simulink model "CDPR_simulation"  (R2021b)
settings: Solver=VariableStepAuto  StartTime=0.0  StopTime=40.0  RelTol=1e-3
values from neighbouring files (symbols this model uses):
  a = [-2.0 2.0 ... (first row only)    [init.m]
  A_p = [0  1   0  0   0  0 ... (first row only)    [init.m]
  b = [-0.05  0.05 ... (first row only)    [init.m]
  B_p = [0     0     0 ... (first row only)    [init.m]
  Clarke = 2/3*[1 -1/2       -1/2 ... (first row only)    [motor_init.m]
  epsilon_1 = 1e-17    [init.m]
  epsilon_2 = 1e-17    [init.m]
  f_max = 60*ones(m,1)    [init.m]
  f_min = 2*ones(m,1)    [init.m]
  f_ref = 0.5*(f_min+f_max)    [init.m]
  fourier_coeff_a = [ 0.08333    0.00000     0.00000 ... (first row only)    [motor_init.m]
  fourier_coeff_b = [-1.23020    0.60792     0.60792 ... (first row only)    [motor_init.m]
  J_m_inv = 1000*1/J_m    (= 41564.487302)    [motor_init.m]
  K_e = 0.052    [motor_init.m]
  k_spring = diag(200*ones(m,1))    [init.m]
  k_spring_inv = inv(k_spring)    [init.m]
  l_0 = inverseKinematics(a, b, x, m)    [init.m]
  L_m = 8.97e-6    (= 8.97e-06)    [motor_init.m]
  m = 4    [init.m]
  n_pole_pairs = n_poles/2    (= 7)    [motor_init.m]
  R_m = 19.00e-3    (= 0.019)    [motor_init.m]
  r_winch = 60.0e-3    (= 0.06)    [init.m]
  tau = 1e-6    (= 1e-06)    [init.m]
  theta_r_0 = (l_0-k_spring_inv*f_ref)/r_winch    [init.m]
  x_0 = [x(1); 0; x(2); 0; x(3);0]    [init.m]
  xi = 2    [init.m]
(part 1 of 2)
settings Model: Creator=Sølve  LastModifiedBy=Sølve

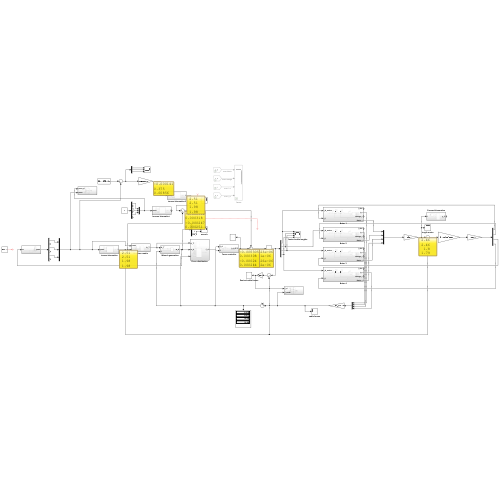
[thumbnail: Simulink's stored preview of the top-level diagram]
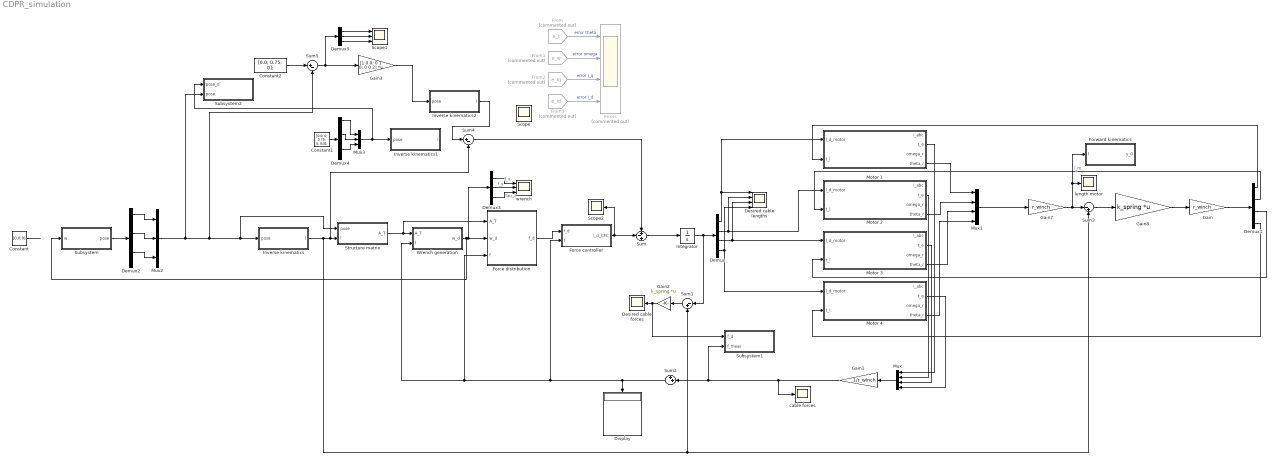
== system CDPR_simulation ==
  Constant : Constant  Value=[0;0;0]
  Constant1 : Constant  Value=[0.0; 0; 0.75; 0; 0;0];
  Constant2 : Constant  Value=[0.0; 0.75; 0];
  Demux : Demux
  Demux1 : Demux
  Demux2 : Demux  Outputs=6
  Demux3 : Demux  Outputs=3
  Demux4 : Demux  Outputs=6
  Demux5 : Demux  Outputs=3
  Desired cable forces : Scope
  Desired cable lengths : Scope  NumInputPorts=4
  Display : Display
      settings: Decimation=3
  Errors : Scope  Commented=on  NumInputPorts=4
  Force controller : Subsystem
  Force distribution : Subsystem
  Forward kinematics : Subsystem
  From : From  Commented=on  GotoTag=e_t  TagVisibility=global
  From1 : From  Commented=on  GotoTag=e_w  TagVisibility=global
  From2 : From  Commented=on  GotoTag=e_iq  TagVisibility=global
  From3 : From  Commented=on  GotoTag=e_id  TagVisibility=global
  Gain : Gain  Gain=r_winch
  Gain1 : Gain  Gain=1/r_winch
  Gain2 : Gain  Gain=k_spring  Multiplication=Matrix(K*u) (u vector)
  Gain3 : Gain  Gain=[1 0 0; 0 1 0; 0 0 2]  Multiplication=Matrix(K*u) (u vector)
  Gain7 : Gain  Gain=r_winch
  Gain8 : Gain  Gain=k_spring  Multiplication=Matrix(K*u) (u vector)
  Integrator : Integrator  InitialCondition=l_0-k_spring_inv*f_ref
  Inverse kinematics : Subsystem
  Inverse kinematics1 : Subsystem
  Inverse kinematics2 : Subsystem
  Motor 1 : Subsystem
  Motor 2 : Subsystem
  Motor 3 : Subsystem
  Motor 4 : Subsystem
  Mux : Mux
  Mux1 : Mux
  Mux2 : Mux  Inputs=3
  Mux3 : Mux  Inputs=3
  Scope : Scope
  Scope1 : Scope  NumInputPorts=3
  Scope2 : Scope
  Structure matrix : Subsystem
  Subsystem : Subsystem
  Subsystem1 : Subsystem
  Subsystem2 : Subsystem
  Sum : Sum  Inputs=+-+
  Sum1 : Sum  Inputs=|-+
  Sum2 : Sum  Inputs=++|
  Sum3 : Sum  Inputs=|-+
  Sum4 : Sum  Inputs=|+-
  Sum5 : Sum  Inputs=|+-
  Wrench generation : Subsystem
  cable forces : Scope
  length motor : Scope
  wrench : Scope  NumInputPorts=3
  wires:
  Mux2/1 -> Subsystem2/2(pose), Sum5/2, Structure matrix/1(pose), Inverse kinematics/1(pose)
  Constant/1 -> ?
  Structure matrix/1(A_T) -> Force distribution/1(A_T), Wrench generation/1(A_T)
  Wrench generation/1(w_d) -> Subsystem/1(w), Force distribution/2(w_d), Demux3/1
  Force controller/1(l_d_CFC) -> Sum/2, Scope2/1
  From3/1 -> Errors/4  "error i_d"
  From2/1 -> Errors/3  "error i_q"
  From/1 -> Errors/1  "error theta"
  From1/1 -> Errors/2  "error omega"
  Sum/1 -> Integrator/1
  Demux/1 -> Desired cable lengths/1, Motor 1/1(l_d_motor)
  Motor 1/4(theta_r) -> Mux1/1
  Sum2/1 -> Force controller/2(f), Force distribution/3(f), Wrench generation/2(f), Display/1
  Demux3/1 -> wrench/1  "f_x"
  Demux3/2 -> wrench/2  "f_y"
  Demux3/3 -> wrench/3  "tau_z"
  Demux/2 -> Motor 2/1(l_d_motor), Desired cable lengths/2
  Mux1/1 -> Gain7/1
  Motor 2/4(theta_r) -> Mux1/2
  Gain7/1 -> length motor/1, Forward kinematics/1(l), Sum3/1  "l_m"
  Motor 3/4(theta_r) -> Mux1/3
  Demux/3 -> Motor 3/1(l_d_motor), Desired cable lengths/3
  Demux/4 -> Motor 4/1(l_d_motor), Desired cable lengths/4
  Motor 4/4(theta_r) -> Mux1/4
  Sum3/1 -> Gain8/1
  Inverse kinematics/1(l) -> Sum1/2, Sum3/2, Sum4/2, Structure matrix/2(l)
  Gain8/1 -> Gain/1
  Gain/1 -> Demux1/1
  Demux1/1 -> Motor 1/2(t_l)
  Demux1/2 -> Motor 2/2(t_l)
  Demux1/3 -> Motor 3/2(t_l)
  Demux1/4 -> Motor 4/2(t_l)
  Motor 1/2(t_e) -> Mux/1
  Motor 2/2(t_e) -> Mux/2
  Motor 3/2(t_e) -> Mux/3
  Motor 4/2(t_e) -> Mux/4
  Mux/1 -> Gain1/1
  Force distribution/1(f_d) -> Force controller/1(f_d)
  Gain1/1 -> cable forces/1, Subsystem1/2(f_meas), Sum2/2
  Integrator/1 -> Sum1/1, Demux/1
  Subsystem/1(pose) -> Demux2/1
  Demux2/1 -> Mux2/1
  Demux2/3 -> Mux2/2
  Demux2/5 -> Mux2/3
  Gain2/1 -> Subsystem1/1(f_d), Desired cable forces/1
  Sum1/1 -> Gain2/1
  Constant1/1 -> Demux4/1
  Inverse kinematics2/1(l) -> Sum4/1
  Sum4/1 -> Sum/1
  Demux4/1 -> Mux3/1
  Demux4/3 -> Mux3/2
  Demux4/5 -> Mux3/3
  Mux3/1 -> Subsystem2/1(pose_d), Inverse kinematics1/1(pose)
  Constant2/1 -> Sum5/1
  Sum5/1 -> Gain3/1, Demux5/1
  Demux5/1 -> Scope1/1
  Demux5/2 -> Scope1/2
  Demux5/3 -> Scope1/3
  Gain3/1 -> Inverse kinematics2/1(pose)
  ? -> ?

== system CDPR_simulation/Force controller ==
  f_d : Inport
  f : Inport  Port=2
  Gain : Gain  Gain=5
  Gain1 : Gain  Gain=k_spring_inv  Multiplication=Matrix(K*u) (u vector)
  Gain2 : Gain  Gain=2
  Integrator : Integrator
  Sum : Sum  Inputs=|+-
  Sum1 : Sum  Inputs=++|
  l_d_CFC : Outport
  wires:
  f_d/1 -> Sum/1
  f/1 -> Sum/2
  Sum/1 -> Integrator/1, Gain/1
  Gain/1 -> Sum1/2
  Gain1/1 -> l_d_CFC/1
  Integrator/1 -> Gain2/1
  Gain2/1 -> ?
  Sum1/1 -> Gain1/1

== system CDPR_simulation/Force distribution ==
  A_T : Inport
  w_d : Inport  Port=2
  f : Inport  Port=3
  Constant : Constant  Commented=on  Value=f_min
  Constant1 : Constant  Commented=on  Value=f_max
  Constant2 : Constant  Value=f_min
  Constant3 : Constant  Value=f_max
  Constant4 : Constant  Value=f_ref
  Constant5 : Constant  Value=m
  Force distribution calculation : MATLAB Function  TreatAsAtomicUnit=on
  MATLAB Function : MATLAB Function  Commented=on  TreatAsAtomicUnit=on
  f_d : Outport
  wires:
  A_T/1 -> Force distribution calculation/1(A_T)
  Force distribution calculation/1(f_d) -> f_d/1
  Constant1/1 -> MATLAB Function/4(f_max)
  Constant/1 -> MATLAB Function/3(f_min)
  w_d/1 -> Force distribution calculation/6(w)
  Constant2/1 -> Force distribution calculation/3(f_min)
  Constant3/1 -> Force distribution calculation/4(f_max)
  Constant4/1 -> Force distribution calculation/5(f_ref)
  Constant5/1 -> Force distribution calculation/7(m)
  f/1 -> Force distribution calculation/2(f)

== system CDPR_simulation/Forward kinematics ==
  l : Inport
  Constant : Constant  Value=b
  Constant1 : Constant  Value=a
  Constant2 : Constant  Value=m
  Constant3 : Constant  Value=tau
  Constant4 : Constant  Value=epsilon_1
  Constant5 : Constant  Value=epsilon_2
  Constant6 : Constant  Value=xi
  MATLAB Function : MATLAB Function  TreatAsAtomicUnit=on
  MATLAB Function1 : MATLAB Function  TreatAsAtomicUnit=on
  y_0 : Outport
  wires:
  l/1 -> MATLAB Function1/3(l), MATLAB Function/4(l)
  Constant/1 -> MATLAB Function1/2(b), MATLAB Function/2(b)
  Constant1/1 -> MATLAB Function1/1(a), MATLAB Function/1(a)
  MATLAB Function1/1(y_0) -> MATLAB Function/3(y_0)
  Constant2/1 -> MATLAB Function/9(m)
  MATLAB Function/1(y_i) -> y_0/1
  Constant3/1 -> MATLAB Function/5(tau)
  Constant5/1 -> MATLAB Function/7(epsilon_2)
  Constant4/1 -> MATLAB Function/6(epsilon_1)
  Constant6/1 -> MATLAB Function/8(xi)

== system CDPR_simulation/Inverse kinematics ==
  pose : Inport
  Constant2 : Constant  Value=m
  Distal anchor points : Constant  Value=b
  Inverse kinematics : MATLAB Function  TreatAsAtomicUnit=on
  Proximal anchor points : Constant  Value=a
  l : Outport
  wires:
  Constant2/1 -> Inverse kinematics/4(m)
  Proximal anchor points/1 -> Inverse kinematics/1(a)
  Inverse kinematics/1(l) -> l/1
  Distal anchor points/1 -> Inverse kinematics/2(b)
  pose/1 -> Inverse kinematics/3(pose)

== system CDPR_simulation/Inverse kinematics1 ==
  pose : Inport
  Constant2 : Constant  Value=m
  Distal anchor points : Constant  Value=b
  Inverse kinematics : MATLAB Function  TreatAsAtomicUnit=on
  Proximal anchor points : Constant  Value=a
  l : Outport
  wires:
  pose/1 -> Inverse kinematics/3(pose)
  Distal anchor points/1 -> Inverse kinematics/2(b)
  Inverse kinematics/1(l) -> l/1
  Proximal anchor points/1 -> Inverse kinematics/1(a)
  Constant2/1 -> Inverse kinematics/4(m)

== system CDPR_simulation/Inverse kinematics2 ==
  pose : Inport
  Constant2 : Constant  Value=m
  Distal anchor points : Constant  Value=b
  Inverse kinematics : MATLAB Function  TreatAsAtomicUnit=on
  Proximal anchor points : Constant  Value=a
  l : Outport
  wires:
  Constant2/1 -> Inverse kinematics/4(m)
  Proximal anchor points/1 -> Inverse kinematics/1(a)
  Inverse kinematics/1(l) -> l/1
  Distal anchor points/1 -> Inverse kinematics/2(b)
  pose/1 -> Inverse kinematics/3(pose)

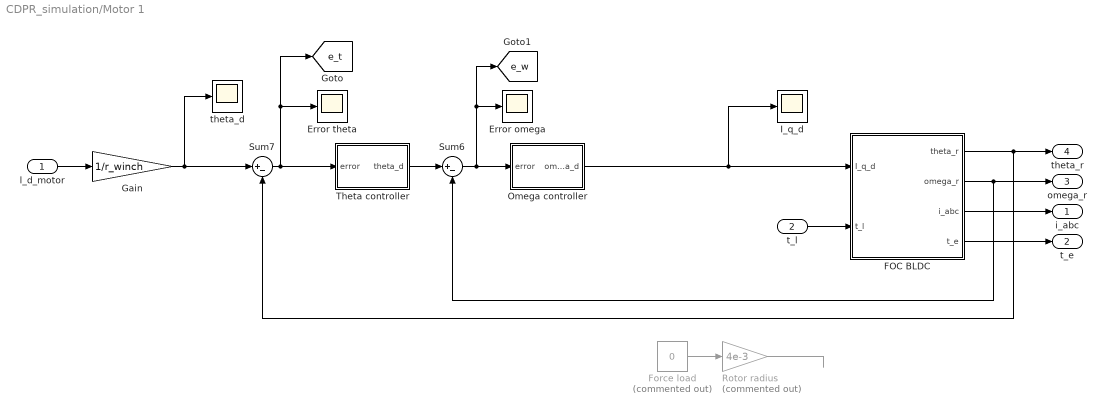
== system CDPR_simulation/Motor 1 ==
  l_d_motor : Inport
  t_l : Inport  Port=2
  Error omega : Scope
  Error theta : Scope
  FOC BLDC : Subsystem
  Force load : Constant  Commented=on  Value=0
  Gain : Gain  Gain=1/r_winch
  I_q_d : Scope
  Omega controller : Subsystem
  Rotor radius : Gain  Commented=on  Gain=4e-3
  Sum6 : Sum  Inputs=|+-
  Sum7 : Sum  Inputs=|+-
  Theta controller : Subsystem
  theta_d : Scope
  i_abc : Outport
  t_e : Outport  Port=2
  omega_r : Outport  Port=3
  theta_r : Outport  Port=4
  tag scope: e_t=global, e_w=global
  wires:
  FOC BLDC/2(omega_r) -> omega_r/1, Sum6/2
  FOC BLDC/3(i_abc) -> i_abc/1
  Sum7/1 -> Theta controller/1(error), [e_t], Error theta/1
  Sum6/1 -> Omega controller/1(error), Error omega/1, [e_w]
  Force load/1 -> Rotor radius/1
  FOC BLDC/1(theta_r) -> theta_r/1, Sum7/2
  Rotor radius/1 -> ?
  Theta controller/1(theta_d) -> Sum6/1
  FOC BLDC/4(t_e) -> t_e/1
  Omega controller/1(omega_d) -> I_q_d/1, FOC BLDC/1(I_q_d)
  l_d_motor/1 -> Gain/1
  t_l/1 -> FOC BLDC/2(t_l)
  Gain/1 -> theta_d/1, Sum7/1

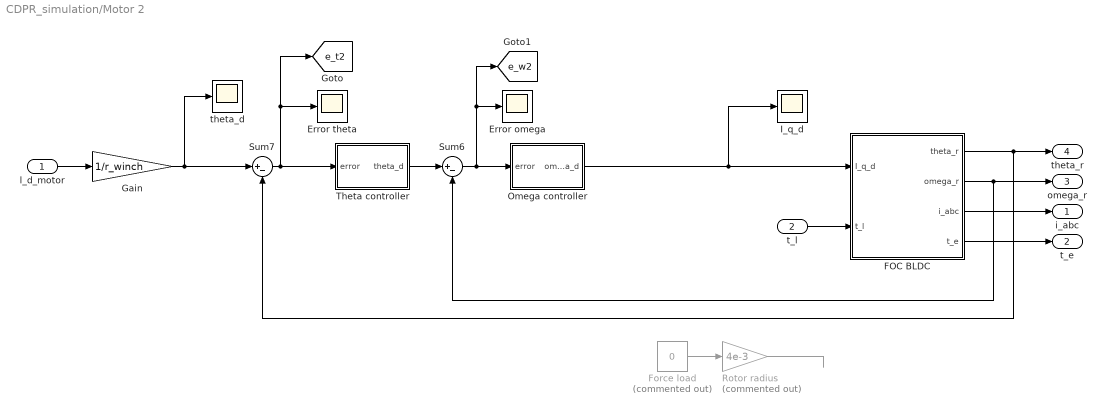
== system CDPR_simulation/Motor 2 ==
  l_d_motor : Inport
  t_l : Inport  Port=2
  Error omega : Scope
  Error theta : Scope
  FOC BLDC : Subsystem
  Force load : Constant  Commented=on  Value=0
  Gain : Gain  Gain=1/r_winch
  I_q_d : Scope
  Omega controller : Subsystem
  Rotor radius : Gain  Commented=on  Gain=4e-3
  Sum6 : Sum  Inputs=|+-
  Sum7 : Sum  Inputs=|+-
  Theta controller : Subsystem
  theta_d : Scope
  i_abc : Outport
  t_e : Outport  Port=2
  omega_r : Outport  Port=3
  theta_r : Outport  Port=4
  tag scope: e_t2=global, e_w2=global
  wires:
  Gain/1 -> Sum7/1, theta_d/1
  t_l/1 -> FOC BLDC/2(t_l)
  l_d_motor/1 -> Gain/1
  Omega controller/1(omega_d) -> FOC BLDC/1(I_q_d), I_q_d/1
  FOC BLDC/4(t_e) -> t_e/1
  Theta controller/1(theta_d) -> Sum6/1
  Rotor radius/1 -> ?
  FOC BLDC/1(theta_r) -> Sum7/2, theta_r/1
  Force load/1 -> Rotor radius/1
  Sum6/1 -> [e_w2], Error omega/1, Omega controller/1(error)
  Sum7/1 -> Error theta/1, [e_t2], Theta controller/1(error)
  FOC BLDC/3(i_abc) -> i_abc/1
  FOC BLDC/2(omega_r) -> Sum6/2, omega_r/1

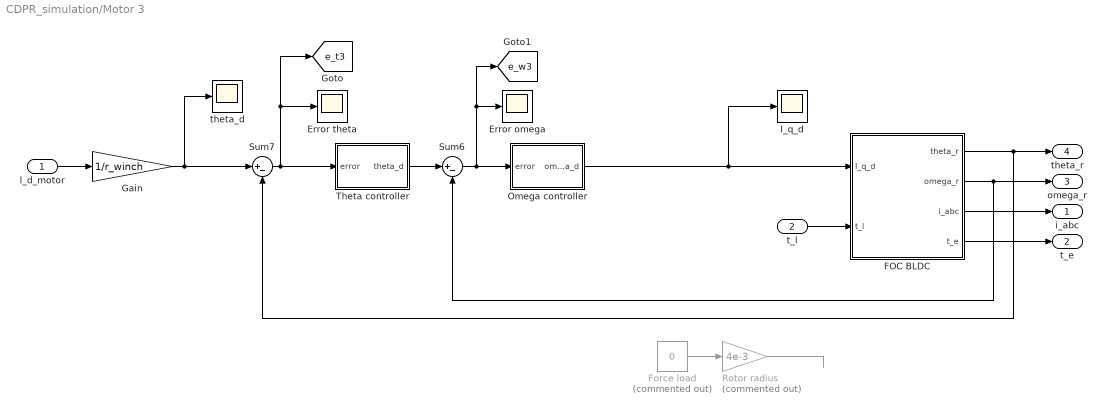
== system CDPR_simulation/Motor 3 ==
  l_d_motor : Inport
  t_l : Inport  Port=2
  Error omega : Scope
  Error theta : Scope
  FOC BLDC : Subsystem
  Force load : Constant  Commented=on  Value=0
  Gain : Gain  Gain=1/r_winch
  I_q_d : Scope
  Omega controller : Subsystem
  Rotor radius : Gain  Commented=on  Gain=4e-3
  Sum6 : Sum  Inputs=|+-
  Sum7 : Sum  Inputs=|+-
  Theta controller : Subsystem
  theta_d : Scope
  i_abc : Outport
  t_e : Outport  Port=2
  omega_r : Outport  Port=3
  theta_r : Outport  Port=4
  tag scope: e_t3=global, e_w3=global
  wires:
  FOC BLDC/2(omega_r) -> omega_r/1, Sum6/2
  FOC BLDC/3(i_abc) -> i_abc/1
  Sum7/1 -> Theta controller/1(error), [e_t3], Error theta/1
  Sum6/1 -> Omega controller/1(error), Error omega/1, [e_w3]
  Force load/1 -> Rotor radius/1
  FOC BLDC/1(theta_r) -> theta_r/1, Sum7/2
  Rotor radius/1 -> ?
  Theta controller/1(theta_d) -> Sum6/1
  FOC BLDC/4(t_e) -> t_e/1
  Omega controller/1(omega_d) -> I_q_d/1, FOC BLDC/1(I_q_d)
  l_d_motor/1 -> Gain/1
  t_l/1 -> FOC BLDC/2(t_l)
  Gain/1 -> theta_d/1, Sum7/1

== system CDPR_simulation/Motor 4 ==
  l_d_motor : Inport
  t_l : Inport  Port=2
  Error omega : Scope
  Error theta : Scope
  FOC BLDC : Subsystem
  Force load : Constant  Commented=on  Value=0
  Gain : Gain  Gain=1/r_winch
  I_q_d : Scope
  Omega controller : Subsystem
  Rotor radius : Gain  Commented=on  Gain=4e-3
  Sum6 : Sum  Inputs=|+-
  Sum7 : Sum  Inputs=|+-
  Theta controller : Subsystem
  theta_d : Scope
  i_abc : Outport
  t_e : Outport  Port=2
  omega_r : Outport  Port=3
  theta_r : Outport  Port=4
  tag scope: e_t4=global, e_w4=global
  wires:
  Gain/1 -> Sum7/1, theta_d/1
  t_l/1 -> FOC BLDC/2(t_l)
  l_d_motor/1 -> Gain/1
  Omega controller/1(omega_d) -> FOC BLDC/1(I_q_d), I_q_d/1
  FOC BLDC/4(t_e) -> t_e/1
  Theta controller/1(theta_d) -> Sum6/1
  Rotor radius/1 -> ?
  FOC BLDC/1(theta_r) -> Sum7/2, theta_r/1
  Force load/1 -> Rotor radius/1
  Sum6/1 -> [e_w4], Error omega/1, Omega controller/1(error)
  Sum7/1 -> Error theta/1, [e_t4], Theta controller/1(error)
  FOC BLDC/3(i_abc) -> i_abc/1
  FOC BLDC/2(omega_r) -> Sum6/2, omega_r/1

== system CDPR_simulation/Structure matrix ==
  pose : Inport
  l : Inport  Port=2
  Constant : Constant  Value=a
  Constant1 : Constant  Value=b
  Constant2 : Constant  Value=m
  MATLAB Function : MATLAB Function  TreatAsAtomicUnit=on
  Structure matrix calculation : MATLAB Function  TreatAsAtomicUnit=on
  A_T : Outport
  wires:
  pose/1 -> Structure matrix calculation/2(pose), MATLAB Function/3(pose)
  Constant1/1 -> Structure matrix calculation/3(b), MATLAB Function/2(b)
  Constant/1 -> MATLAB Function/1(a)
  MATLAB Function/1(u) -> Structure matrix calculation/1(u)
  Structure matrix calculation/1(A_T) -> A_T/1
  l/1 -> MATLAB Function/4(l_ik)
  Constant2/1 -> Structure matrix calculation/4(m), MATLAB Function/5(m)

== system CDPR_simulation/Subsystem ==
  w : Inport
  Demux : Demux  Outputs=6
  Gain : Gain  Gain=B_p  Multiplication=Matrix(K*u) (u vector)
  Gain1 : Gain  Gain=A_p  Multiplication=Matrix(K*u) (u vector)
  Integrator : Integrator  InitialCondition=x_0
  Mux : Mux  Inputs=6
  Scope : Scope  NumInputPorts=3
  Sum : Sum  Inputs=|++
  XY Graph : Record  FileSettingsInternal="{\"entries\":[{\"content\":{\"excelSettings\":{\"content\":{},\"type\":\"Streamout.ExcelSettings\"}},\"type\":\"Streamout.FileSettingStorage\",\"uuid\":\"53abfe96-87d4-4a9b-ba96-94057390cc17\"}],\"packageUris\":[\"http://schema.mathworks.com/mf0/streamout_blocks/R2020a\"],\"version\":\"1.0\"}"  Layout=[1 1]  SignalsInternal="{\"entries\":[{\"content\":{\"signals\":[{\"content\":{\"blockPath\":[\"CDPR_simulation/Subsystem/XY Graph\"],\"channel\":[],\"dimensions\":[1],\"domain\":\"CDPR_simulation/Subsystem/XY Graph\",\"lineColor\":\"#a2142f\",\"plots\":[1],\"port\":1,\"sid\":[\"\"],\"signalID\":17344,\"signalName\":\"Demux:1\"},\"type\":\"RecordBlkView.Signal\",\"uuid\":\"32875e08-411f-4073-9301-21440afacdc0\"},{\"content\":{\"blockPath\":[\"CDPR_simulation/Subsystem/XY Graph\"],\"channel\":[],\"dimensions\":[1],\"domain\":\"CDPR_simulation/Subsystem/XY Graph\",\"lineColor\":\"#139fff\",\"plots\":[1],\"port\":2,\"sid\":[\"\"],\"signalID\":17348,\"signalName\":\"Demux:3\"},\"type\":\"RecordBlkView.Signal\",\"uuid\":\"bdc768ac-4432-491c-a3b0-f805c164fc47\"}]},\"type\":\"RecordBlkView.InputSignals\",\"uuid\":\"dc717eb6-7a39-403c-b8e2-f99afc544a76\"}],\"packageUris\":[\"http://schema.mathworks.com/mf0/streamout_blocks/R2020a\"],\"version\":\"1.0\"}"  VisualizationBindings="{\"xyplotplugin\":{\"info\":[{\"series\":[{\"bindingParametersList\":[{\"parameter\":\"X-Axis\",\"signalID\":17344,\"signalName\":\"Demux:1\"},{\"parameter\":\"Y-Axis\",\"signalID\":17348,\"signalName\":\"Demux:3\"}],\"seriesID\":4472}],\"subplotID\":1}]}}"  CompatibilityTag=XY
  pose : Outport
  wires:
  w/1 -> Gain/1
  Gain/1 -> Sum/1
  Sum/1 -> Integrator/1
  Gain1/1 -> Sum/2
  Integrator/1 -> Demux/1, Gain1/1
  Demux/1 -> XY Graph/1, Scope/1, Mux/1
  Demux/3 -> Scope/2, XY Graph/2, Mux/3
  Demux/5 -> Scope/3, Mux/5
  Mux/1 -> pose/1
  Demux/2 -> Mux/2
  Demux/4 -> Mux/4
  Demux/6 -> Mux/6

== system CDPR_simulation/Subsystem1 ==
  f_d : Inport
  f_meas : Inport  Port=2
  Demux : Demux
  Demux1 : Demux
  Desired v. measured cable forces : Scope  NumInputPorts=4
  Mux{,1..3} (4 alike) : Mux  Inputs=2
  wires:
  f_d/1 -> Demux/1
  f_meas/1 -> Demux1/1
  Demux/1 -> Mux/1  "Desired force cable 1"
  Demux1/1 -> Mux/2  "Measured force cable 1"
  Demux/2 -> Mux1/1  "Desired force cable 2"
  Demux1/2 -> Mux1/2  "Measured force cable 2"
  Demux/3 -> Mux2/1  "Desired force cable 3"
  Demux1/3 -> Mux2/2  "Measured force cable 3"
  Demux/4 -> Mux3/1  "Desired force cable 4"
  Demux1/4 -> Mux3/2  "Measured force cable 4"
  Mux/1 -> Desired v. measured cable forces/1
  Mux1/1 -> Desired v. measured cable forces/2
  Mux2/1 -> Desired v. measured cable forces/3
  Mux3/1 -> Desired v. measured cable forces/4

== system CDPR_simulation/Subsystem2 ==
  pose_d : Inport
  pose : Inport  Port=2
  Demux : Demux  Outputs=3
  Demux1 : Demux  Outputs=3
  Desired v. actual pose : Scope  NumInputPorts=3
  Mux : Mux  Inputs=2
  Mux1 : Mux  Inputs=2
  Mux2 : Mux  Inputs=2
  wires:
  pose_d/1 -> Demux/1
  pose/1 -> Demux1/1
  Demux/1 -> Mux/1  "Desired x-coord"
  Demux1/1 -> Mux/2  "Actual x-coord"
  Demux/2 -> Mux1/1  "Desired y-coord"
  Demux1/2 -> Mux1/2  "Actual y-coord"
  Demux1/3 -> Mux2/2  "Actual angle"
  Demux/3 -> Mux2/1  "Desired angle"
  Mux/1 -> Desired v. actual pose/1
  Mux1/1 -> Desired v. actual pose/2
  Mux2/1 -> Desired v. actual pose/3

== system CDPR_simulation/Wrench generation ==
  A_T : Inport
  f : Inport  Port=2
  Gain : Gain
  Matrix Multiply : Product  Multiplication=Matrix(*)
  w_d : Outport
  wires:
  A_T/1 -> Gain/1
  f/1 -> Matrix Multiply/2
  Gain/1 -> Matrix Multiply/1
  Matrix Multiply/1 -> w_d/1

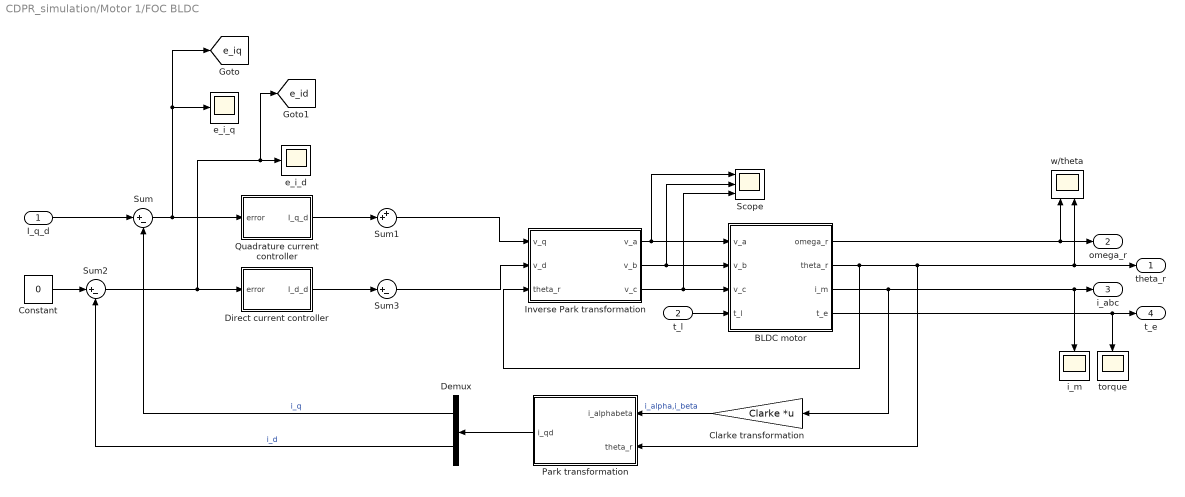
== system CDPR_simulation/Motor 1/FOC BLDC ==
  I_q_d : Inport
  t_l : Inport  Port=2
  BLDC motor : Subsystem
  Clarke transformation : Gain  Gain=Clarke  Multiplication=Matrix(K*u) (u vector)
  Constant : Constant  Value=0
  Demux : Demux  Outputs=2
  Direct current controller : Subsystem
  Inverse Park transformation : MATLAB Function  TreatAsAtomicUnit=on
  Park transformation : MATLAB Function  TreatAsAtomicUnit=on
  Quadrature current controller : Subsystem
  Scope : Scope  NumInputPorts=3
  Sum : Sum  Inputs=|+-
  Sum1 : Sum  Inputs=++|
  Sum2 : Sum  Inputs=|+-
  Sum3 : Sum  Inputs=|+-
  e_i_d : Scope
  e_i_q : Scope
  i_m : Scope
  torque : Scope
  w/theta : Scope  NumInputPorts=2
  theta_r : Outport
  omega_r : Outport  Port=2
  i_abc : Outport  Port=3
  t_e : Outport  Port=4
  tag scope: e_id=global, e_iq=global
  wires:
  Sum/1 -> Quadrature current controller/1(error), [e_iq], e_i_q/1
  Quadrature current controller/1(I_q_d) -> Sum1/2
  Constant/1 -> Sum2/1
  Sum2/1 -> Direct current controller/1(error), [e_id], e_i_d/1
  Direct current controller/1(I_d_d) -> Sum3/1
  Sum1/1 -> Inverse Park transformation/1(v_q)
  Sum3/1 -> Inverse Park transformation/2(v_d)
  Inverse Park transformation/1(v_a) -> Scope/1, BLDC motor/1(v_a)
  Inverse Park transformation/2(v_b) -> Scope/2, BLDC motor/2(v_b)
  Inverse Park transformation/3(v_c) -> Scope/3, BLDC motor/3(v_c)
  t_l/1 -> BLDC motor/4(t_l)
  BLDC motor/1(omega_r) -> omega_r/1, w/theta/1
  Clarke transformation/1 -> Park transformation/1(i_alphabeta)  "i_alpha,i_beta"
  BLDC motor/2(theta_r) -> Park transformation/2(theta_r), theta_r/1, w/theta/2, Inverse Park transformation/3(theta_r)
  Park transformation/1(i_qd) -> Demux/1
  Demux/1 -> Sum/2  "i_q"
  Demux/2 -> Sum2/2  "i_d"
  BLDC motor/3(i_m) -> i_m/1, i_abc/1, Clarke transformation/1
  BLDC motor/4(t_e) -> torque/1, t_e/1
  I_q_d/1 -> Sum/1

== system CDPR_simulation/Motor 1/Omega controller ==
  error : Inport
  Gain : Gain  Gain=30
  Gain1 : Gain  Gain=120
  Gain2 : Gain  Gain=30
  Gain3 : Gain  Gain=70
  Integrator : Integrator
  Sum : Sum  Inputs=++|
  omega_d : Outport
  wires:
  Sum/1 -> omega_d/1
  Gain/1 -> Sum/1
  Gain1/1 -> Sum/2
  Integrator/1 -> Gain1/1
  error/1 -> Integrator/1, Gain/1

== system CDPR_simulation/Motor 1/Theta controller ==
  error : Inport
  Gain : Gain  Gain=10
  Gain1 : Gain  Gain=30
  Gain2 : Gain  Gain=0.2
  Gain3 : Gain  Gain=15
  Integrator : Integrator
  Sum : Sum  Inputs=++|
  theta_d : Outport
  wires:
  error/1 -> Gain/1, Integrator/1
  Integrator/1 -> Gain1/1
  Gain1/1 -> Sum/2
  Gain/1 -> Sum/1
  Sum/1 -> theta_d/1

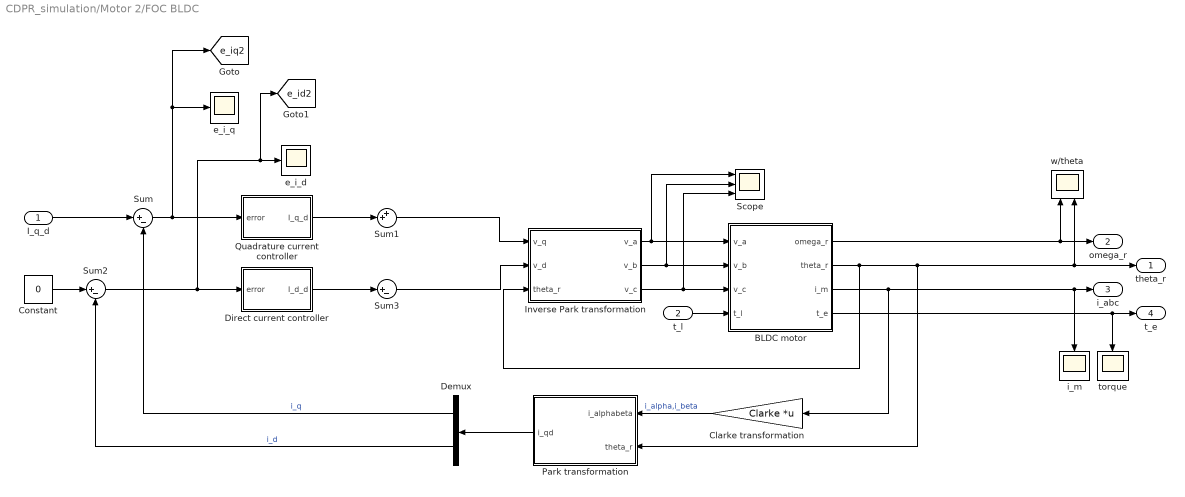
== system CDPR_simulation/Motor 2/FOC BLDC ==
  I_q_d : Inport
  t_l : Inport  Port=2
  BLDC motor : Subsystem
  Clarke transformation : Gain  Gain=Clarke  Multiplication=Matrix(K*u) (u vector)
  Constant : Constant  Value=0
  Demux : Demux  Outputs=2
  Direct current controller : Subsystem
  Inverse Park transformation : MATLAB Function  TreatAsAtomicUnit=on
  Park transformation : MATLAB Function  TreatAsAtomicUnit=on
  Quadrature current controller : Subsystem
  Scope : Scope  NumInputPorts=3
  Sum : Sum  Inputs=|+-
  Sum1 : Sum  Inputs=++|
  Sum2 : Sum  Inputs=|+-
  Sum3 : Sum  Inputs=|+-
  e_i_d : Scope
  e_i_q : Scope
  i_m : Scope
  torque : Scope
  w/theta : Scope  NumInputPorts=2
  theta_r : Outport
  omega_r : Outport  Port=2
  i_abc : Outport  Port=3
  t_e : Outport  Port=4
  tag scope: e_id2=global, e_iq2=global
  wires:
  I_q_d/1 -> Sum/1
  BLDC motor/4(t_e) -> t_e/1, torque/1
  BLDC motor/3(i_m) -> Clarke transformation/1, i_abc/1, i_m/1
  Demux/2 -> Sum2/2  "i_d"
  Demux/1 -> Sum/2  "i_q"
  Park transformation/1(i_qd) -> Demux/1
  BLDC motor/2(theta_r) -> Inverse Park transformation/3(theta_r), w/theta/2, theta_r/1, Park transformation/2(theta_r)
  Clarke transformation/1 -> Park transformation/1(i_alphabeta)  "i_alpha,i_beta"
  BLDC motor/1(omega_r) -> w/theta/1, omega_r/1
  t_l/1 -> BLDC motor/4(t_l)
  Inverse Park transformation/3(v_c) -> BLDC motor/3(v_c), Scope/3
  Inverse Park transformation/2(v_b) -> BLDC motor/2(v_b), Scope/2
  Inverse Park transformation/1(v_a) -> BLDC motor/1(v_a), Scope/1
  Sum3/1 -> Inverse Park transformation/2(v_d)
  Sum1/1 -> Inverse Park transformation/1(v_q)
  Direct current controller/1(I_d_d) -> Sum3/1
  Sum2/1 -> e_i_d/1, [e_id2], Direct current controller/1(error)
  Constant/1 -> Sum2/1
  Quadrature current controller/1(I_q_d) -> Sum1/2
  Sum/1 -> e_i_q/1, [e_iq2], Quadrature current controller/1(error)

== system CDPR_simulation/Motor 2/Omega controller ==
  error : Inport
  Gain : Gain  Gain=30
  Gain1 : Gain  Gain=120
  Gain2 : Gain  Gain=30
  Gain3 : Gain  Gain=70
  Integrator : Integrator
  Sum : Sum  Inputs=++|
  omega_d : Outport
  wires:
  error/1 -> Gain/1, Integrator/1
  Integrator/1 -> Gain1/1
  Gain1/1 -> Sum/2
  Gain/1 -> Sum/1
  Sum/1 -> omega_d/1

== system CDPR_simulation/Motor 2/Theta controller ==
  error : Inport
  Gain : Gain  Gain=10
  Gain1 : Gain  Gain=30
  Gain2 : Gain  Gain=0.2
  Gain3 : Gain  Gain=15
  Integrator : Integrator
  Sum : Sum  Inputs=++|
  theta_d : Outport
  wires:
  Sum/1 -> theta_d/1
  Gain/1 -> Sum/1
  Gain1/1 -> Sum/2
  Integrator/1 -> Gain1/1
  error/1 -> Integrator/1, Gain/1

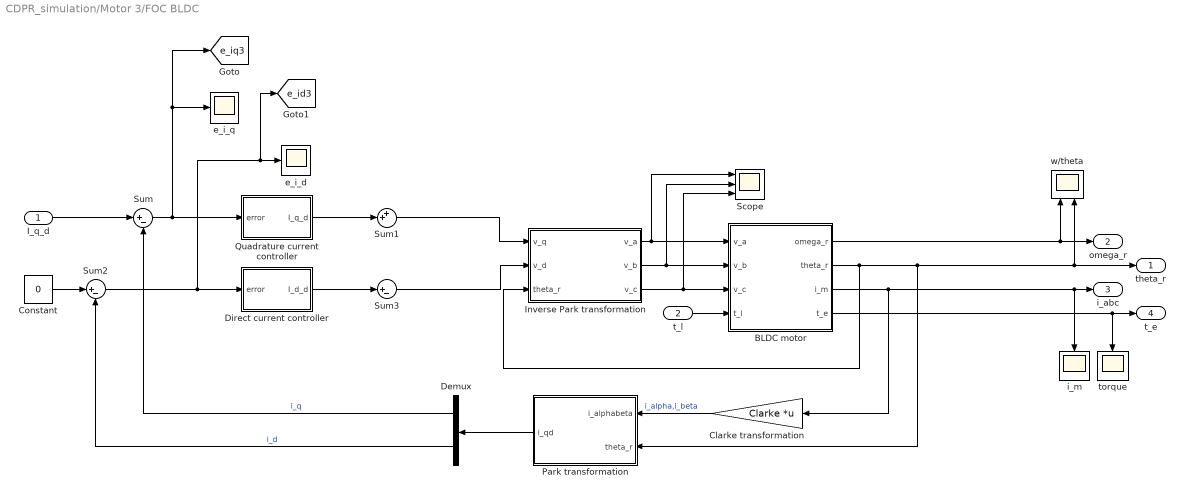
== system CDPR_simulation/Motor 3/FOC BLDC ==
  I_q_d : Inport
  t_l : Inport  Port=2
  BLDC motor : Subsystem
  Clarke transformation : Gain  Gain=Clarke  Multiplication=Matrix(K*u) (u vector)
  Constant : Constant  Value=0
  Demux : Demux  Outputs=2
  Direct current controller : Subsystem
  Inverse Park transformation : MATLAB Function  TreatAsAtomicUnit=on
  Park transformation : MATLAB Function  TreatAsAtomicUnit=on
  Quadrature current controller : Subsystem
  Scope : Scope  NumInputPorts=3
  Sum : Sum  Inputs=|+-
  Sum1 : Sum  Inputs=++|
  Sum2 : Sum  Inputs=|+-
  Sum3 : Sum  Inputs=|+-
  e_i_d : Scope
  e_i_q : Scope
  i_m : Scope
  torque : Scope
  w/theta : Scope  NumInputPorts=2
  theta_r : Outport
  omega_r : Outport  Port=2
  i_abc : Outport  Port=3
  t_e : Outport  Port=4
  tag scope: e_id3=global, e_iq3=global
  wires:
  Sum/1 -> Quadrature current controller/1(error), [e_iq3], e_i_q/1
  Quadrature current controller/1(I_q_d) -> Sum1/2
  Constant/1 -> Sum2/1
  Sum2/1 -> Direct current controller/1(error), [e_id3], e_i_d/1
  Direct current controller/1(I_d_d) -> Sum3/1
  Sum1/1 -> Inverse Park transformation/1(v_q)
  Sum3/1 -> Inverse Park transformation/2(v_d)
  Inverse Park transformation/1(v_a) -> Scope/1, BLDC motor/1(v_a)
  Inverse Park transformation/2(v_b) -> Scope/2, BLDC motor/2(v_b)
  Inverse Park transformation/3(v_c) -> Scope/3, BLDC motor/3(v_c)
  t_l/1 -> BLDC motor/4(t_l)
  BLDC motor/1(omega_r) -> omega_r/1, w/theta/1
  Clarke transformation/1 -> Park transformation/1(i_alphabeta)  "i_alpha,i_beta"
  BLDC motor/2(theta_r) -> Park transformation/2(theta_r), theta_r/1, w/theta/2, Inverse Park transformation/3(theta_r)
  Park transformation/1(i_qd) -> Demux/1
  Demux/1 -> Sum/2  "i_q"
  Demux/2 -> Sum2/2  "i_d"
  BLDC motor/3(i_m) -> i_m/1, i_abc/1, Clarke transformation/1
  BLDC motor/4(t_e) -> torque/1, t_e/1
  I_q_d/1 -> Sum/1

== system CDPR_simulation/Motor 3/Omega controller ==
  error : Inport
  Gain : Gain  Gain=30
  Gain1 : Gain  Gain=120
  Gain2 : Gain  Gain=30
  Gain3 : Gain  Gain=70
  Integrator : Integrator
  Sum : Sum  Inputs=++|
  omega_d : Outport
  wires:
  Sum/1 -> omega_d/1
  Gain/1 -> Sum/1
  Gain1/1 -> Sum/2
  Integrator/1 -> Gain1/1
  error/1 -> Integrator/1, Gain/1

== system CDPR_simulation/Motor 3/Theta controller ==
  error : Inport
  Gain : Gain  Gain=10
  Gain1 : Gain  Gain=30
  Gain2 : Gain  Gain=0.2
  Gain3 : Gain  Gain=15
  Integrator : Integrator
  Sum : Sum  Inputs=++|
  theta_d : Outport
  wires:
  error/1 -> Gain/1, Integrator/1
  Integrator/1 -> Gain1/1
  Gain1/1 -> Sum/2
  Gain/1 -> Sum/1
  Sum/1 -> theta_d/1

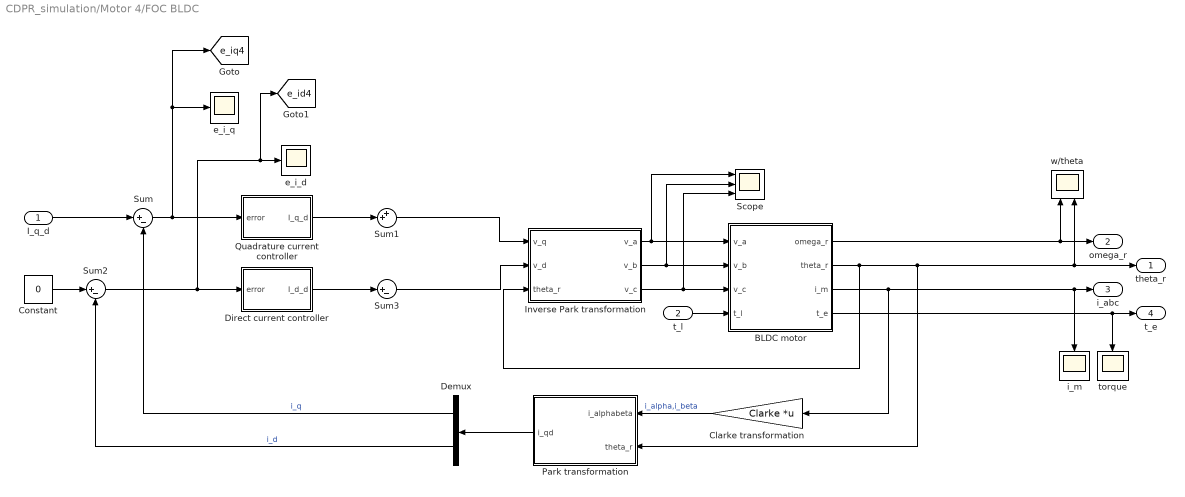
== system CDPR_simulation/Motor 4/FOC BLDC ==
  I_q_d : Inport
  t_l : Inport  Port=2
  BLDC motor : Subsystem
  Clarke transformation : Gain  Gain=Clarke  Multiplication=Matrix(K*u) (u vector)
  Constant : Constant  Value=0
  Demux : Demux  Outputs=2
  Direct current controller : Subsystem
  Inverse Park transformation : MATLAB Function  TreatAsAtomicUnit=on
  Park transformation : MATLAB Function  TreatAsAtomicUnit=on
  Quadrature current controller : Subsystem
  Scope : Scope  NumInputPorts=3
  Sum : Sum  Inputs=|+-
  Sum1 : Sum  Inputs=++|
  Sum2 : Sum  Inputs=|+-
  Sum3 : Sum  Inputs=|+-
  e_i_d : Scope
  e_i_q : Scope
  i_m : Scope
  torque : Scope
  w/theta : Scope  NumInputPorts=2
  theta_r : Outport
  omega_r : Outport  Port=2
  i_abc : Outport  Port=3
  t_e : Outport  Port=4
  tag scope: e_id4=global, e_iq4=global
  wires:
  I_q_d/1 -> Sum/1
  BLDC motor/4(t_e) -> t_e/1, torque/1
  BLDC motor/3(i_m) -> Clarke transformation/1, i_abc/1, i_m/1
  Demux/2 -> Sum2/2  "i_d"
  Demux/1 -> Sum/2  "i_q"
  Park transformation/1(i_qd) -> Demux/1
  BLDC motor/2(theta_r) -> Inverse Park transformation/3(theta_r), w/theta/2, theta_r/1, Park transformation/2(theta_r)
  Clarke transformation/1 -> Park transformation/1(i_alphabeta)  "i_alpha,i_beta"
  BLDC motor/1(omega_r) -> w/theta/1, omega_r/1
  t_l/1 -> BLDC motor/4(t_l)
  Inverse Park transformation/3(v_c) -> BLDC motor/3(v_c), Scope/3
  Inverse Park transformation/2(v_b) -> BLDC motor/2(v_b), Scope/2
  Inverse Park transformation/1(v_a) -> BLDC motor/1(v_a), Scope/1
  Sum3/1 -> Inverse Park transformation/2(v_d)
  Sum1/1 -> Inverse Park transformation/1(v_q)
  Direct current controller/1(I_d_d) -> Sum3/1
  Sum2/1 -> e_i_d/1, [e_id4], Direct current controller/1(error)
  Constant/1 -> Sum2/1
  Quadrature current controller/1(I_q_d) -> Sum1/2
  Sum/1 -> e_i_q/1, [e_iq4], Quadrature current controller/1(error)

== system CDPR_simulation/Motor 4/Omega controller ==
  error : Inport
  Gain : Gain  Gain=30
  Gain1 : Gain  Gain=120
  Gain2 : Gain  Gain=30
  Gain3 : Gain  Gain=70
  Integrator : Integrator
  Sum : Sum  Inputs=++|
  omega_d : Outport
  wires:
  error/1 -> Gain/1, Integrator/1
  Integrator/1 -> Gain1/1
  Gain1/1 -> Sum/2
  Gain/1 -> Sum/1
  Sum/1 -> omega_d/1

== system CDPR_simulation/Motor 4/Theta controller ==
  error : Inport
  Gain : Gain  Gain=10
  Gain1 : Gain  Gain=30
  Gain2 : Gain  Gain=0.2
  Gain3 : Gain  Gain=15
  Integrator : Integrator
  Sum : Sum  Inputs=++|
  theta_d : Outport
  wires:
  Sum/1 -> theta_d/1
  Gain/1 -> Sum/1
  Gain1/1 -> Sum/2
  Integrator/1 -> Gain1/1
  error/1 -> Integrator/1, Gain/1

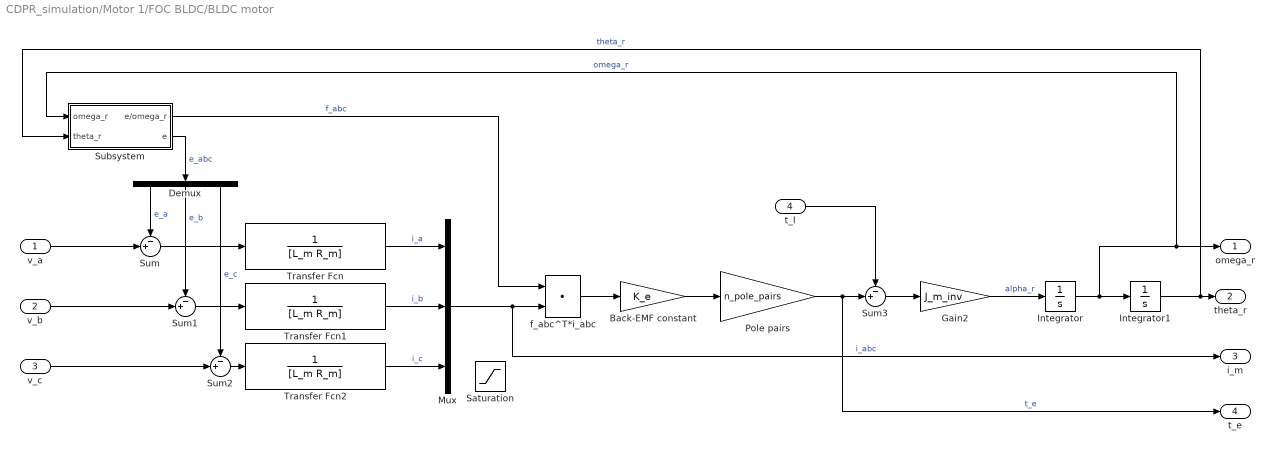
== system CDPR_simulation/Motor 1/FOC BLDC/BLDC motor ==
  v_a : Inport
  v_b : Inport  Port=2
  v_c : Inport  Port=3
  t_l : Inport  Port=4
  Back-EMF constant : Gain  Gain=K_e
  Demux : Demux  Outputs=3
  Gain2 : Gain  Gain=J_m_inv
  Integrator : Integrator  InitialCondition=0.001
  Integrator1 : Integrator  InitialCondition=theta_r_0(1)
  Mux : Mux  Inputs=3
  Pole pairs : Gain  Gain=n_pole_pairs
  Saturation : Saturate  UpperLimit=20  LowerLimit=20
  Subsystem : Subsystem
  Sum{,1..3} (4 alike) : Sum  Inputs=-+|
  Transfer Fcn : TransferFcn  Denominator=[L_m R_m]
  Transfer Fcn1 : TransferFcn  Denominator=[L_m R_m]
  Transfer Fcn2 : TransferFcn  Denominator=[L_m R_m]
  f_abc^T*i_abc : DotProduct  InputSameDT=on  OutDataTypeStr=Inherit: Inherit via internal rule
  omega_r : Outport
  theta_r : Outport  Port=2
  i_m : Outport  Port=3
  t_e : Outport  Port=4
  wires:
  v_a/1 -> Sum/2
  v_b/1 -> Sum1/2
  v_c/1 -> Sum2/2
  Demux/1 -> Sum/1  "e_a"
  Demux/2 -> Sum1/1  "e_b"
  Demux/3 -> Sum2/1  "e_c"
  Subsystem/2(e) -> Demux/1  "e_abc"
  Sum/1 -> Transfer Fcn/1
  Sum1/1 -> Transfer Fcn1/1
  Sum2/1 -> Transfer Fcn2/1
  Transfer Fcn2/1 -> Mux/3  "i_c"
  Transfer Fcn1/1 -> Mux/2  "i_b"
  Transfer Fcn/1 -> Mux/1  "i_a"
  Subsystem/1(e/omega_r) -> f_abc^T*i_abc/1  "f_abc"
  Sum3/1 -> Gain2/1
  f_abc^T*i_abc/1 -> Back-EMF constant/1
  Back-EMF constant/1 -> Pole pairs/1
  t_l/1 -> Sum3/1
  Gain2/1 -> Integrator/1  "alpha_r"
  Integrator/1 -> Subsystem/1(omega_r), omega_r/1, Integrator1/1  "omega_r"
  Integrator1/1 -> Subsystem/2(theta_r), theta_r/1  "theta_r"
  Pole pairs/1 -> t_e/1, Sum3/2  "t_e"
  Mux/1 -> f_abc^T*i_abc/2, i_m/1  "i_abc"

== system CDPR_simulation/Motor 1/FOC BLDC/Direct current controller ==
  error : Inport
  Gain : Gain  Gain=100
  Gain1 : Gain  Gain=70
  Integrator : Integrator
  Sum : Sum  Inputs=++|
  I_d_d : Outport
  wires:
  error/1 -> Gain/1, Integrator/1
  Integrator/1 -> Gain1/1
  Gain1/1 -> Sum/2
  Gain/1 -> Sum/1
  Sum/1 -> I_d_d/1

== system CDPR_simulation/Motor 1/FOC BLDC/Quadrature current controller ==
  error : Inport
  Gain : Gain  Gain=35
  Gain1 : Gain  Gain=50
  Integrator : Integrator
  Sum : Sum  Inputs=++|
  I_q_d : Outport
  wires:
  Sum/1 -> I_q_d/1
  Gain/1 -> Sum/1
  Gain1/1 -> Sum/2
  Integrator/1 -> Gain1/1
  error/1 -> Integrator/1, Gain/1

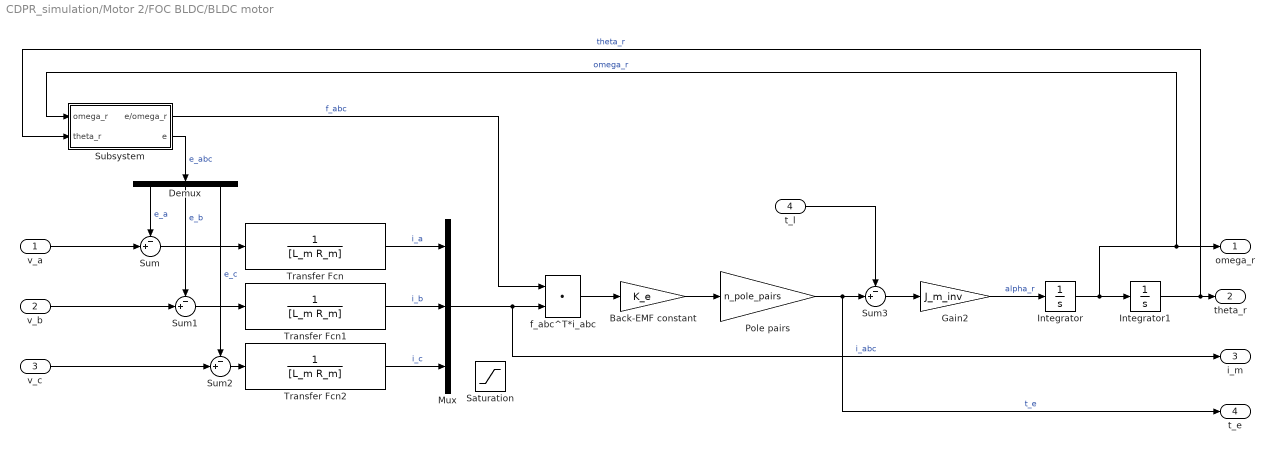
== system CDPR_simulation/Motor 2/FOC BLDC/BLDC motor ==
  v_a : Inport
  v_b : Inport  Port=2
  v_c : Inport  Port=3
  t_l : Inport  Port=4
  Back-EMF constant : Gain  Gain=K_e
  Demux : Demux  Outputs=3
  Gain2 : Gain  Gain=J_m_inv
  Integrator : Integrator  InitialCondition=0.001
  Integrator1 : Integrator  InitialCondition=theta_r_0(2)
  Mux : Mux  Inputs=3
  Pole pairs : Gain  Gain=n_pole_pairs
  Saturation : Saturate  UpperLimit=20  LowerLimit=20
  Subsystem : Subsystem
  Sum{,1..3} (4 alike) : Sum  Inputs=-+|
  Transfer Fcn : TransferFcn  Denominator=[L_m R_m]
  Transfer Fcn1 : TransferFcn  Denominator=[L_m R_m]
  Transfer Fcn2 : TransferFcn  Denominator=[L_m R_m]
  f_abc^T*i_abc : DotProduct  InputSameDT=on  OutDataTypeStr=Inherit: Inherit via internal rule
  omega_r : Outport
  theta_r : Outport  Port=2
  i_m : Outport  Port=3
  t_e : Outport  Port=4
  wires:
  Mux/1 -> i_m/1, f_abc^T*i_abc/2  "i_abc"
  Pole pairs/1 -> Sum3/2, t_e/1  "t_e"
  Integrator1/1 -> theta_r/1, Subsystem/2(theta_r)  "theta_r"
  Integrator/1 -> Integrator1/1, omega_r/1, Subsystem/1(omega_r)  "omega_r"
  Gain2/1 -> Integrator/1  "alpha_r"
  t_l/1 -> Sum3/1
  Back-EMF constant/1 -> Pole pairs/1
  f_abc^T*i_abc/1 -> Back-EMF constant/1
  Sum3/1 -> Gain2/1
  Subsystem/1(e/omega_r) -> f_abc^T*i_abc/1  "f_abc"
  Transfer Fcn/1 -> Mux/1  "i_a"
  Transfer Fcn1/1 -> Mux/2  "i_b"
  Transfer Fcn2/1 -> Mux/3  "i_c"
  Sum2/1 -> Transfer Fcn2/1
  Sum1/1 -> Transfer Fcn1/1
  Sum/1 -> Transfer Fcn/1
  Subsystem/2(e) -> Demux/1  "e_abc"
  Demux/3 -> Sum2/1  "e_c"
  Demux/2 -> Sum1/1  "e_b"
  Demux/1 -> Sum/1  "e_a"
  v_c/1 -> Sum2/2
  v_b/1 -> Sum1/2
  v_a/1 -> Sum/2

== system CDPR_simulation/Motor 2/FOC BLDC/Direct current controller ==
  error : Inport
  Gain : Gain  Gain=100
  Gain1 : Gain  Gain=70
  Integrator : Integrator
  Sum : Sum  Inputs=++|
  I_d_d : Outport
  wires:
  Sum/1 -> I_d_d/1
  Gain/1 -> Sum/1
  Gain1/1 -> Sum/2
  Integrator/1 -> Gain1/1
  error/1 -> Integrator/1, Gain/1

== system CDPR_simulation/Motor 2/FOC BLDC/Quadrature current controller ==
  error : Inport
  Gain : Gain  Gain=35
  Gain1 : Gain  Gain=50
  Integrator : Integrator
  Sum : Sum  Inputs=++|
  I_q_d : Outport
  wires:
  error/1 -> Gain/1, Integrator/1
  Integrator/1 -> Gain1/1
  Gain1/1 -> Sum/2
  Gain/1 -> Sum/1
  Sum/1 -> I_q_d/1

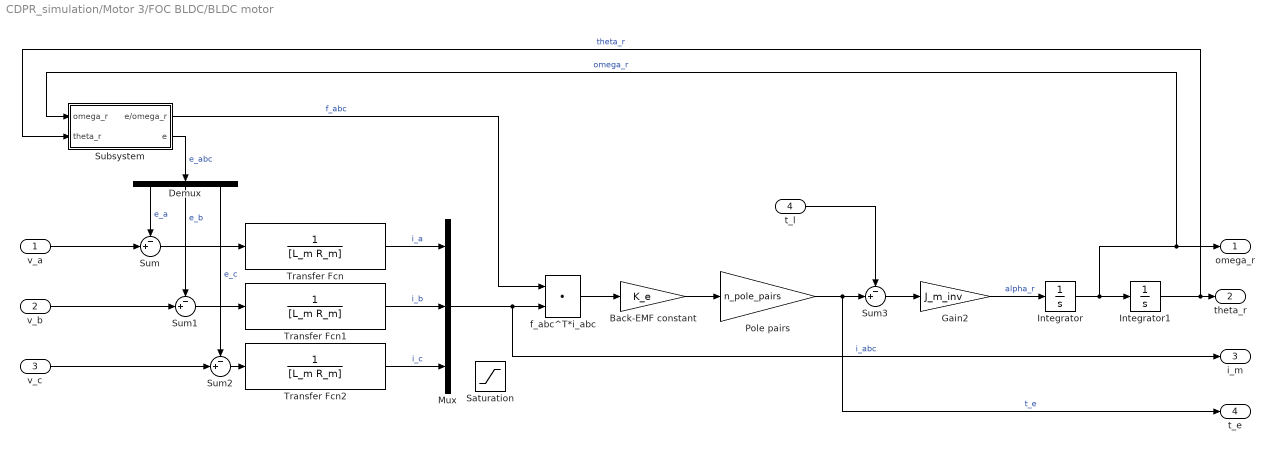
== system CDPR_simulation/Motor 3/FOC BLDC/BLDC motor ==
  v_a : Inport
  v_b : Inport  Port=2
  v_c : Inport  Port=3
  t_l : Inport  Port=4
  Back-EMF constant : Gain  Gain=K_e
  Demux : Demux  Outputs=3
  Gain2 : Gain  Gain=J_m_inv
  Integrator : Integrator  InitialCondition=0.001
  Integrator1 : Integrator  InitialCondition=theta_r_0(3)
  Mux : Mux  Inputs=3
  Pole pairs : Gain  Gain=n_pole_pairs
  Saturation : Saturate  UpperLimit=20  LowerLimit=20
  Subsystem : Subsystem
  Sum{,1..3} (4 alike) : Sum  Inputs=-+|
  Transfer Fcn : TransferFcn  Denominator=[L_m R_m]
  Transfer Fcn1 : TransferFcn  Denominator=[L_m R_m]
  Transfer Fcn2 : TransferFcn  Denominator=[L_m R_m]
  f_abc^T*i_abc : DotProduct  InputSameDT=on  OutDataTypeStr=Inherit: Inherit via internal rule
  omega_r : Outport
  theta_r : Outport  Port=2
  i_m : Outport  Port=3
  t_e : Outport  Port=4
  wires:
  v_a/1 -> Sum/2
  v_b/1 -> Sum1/2
  v_c/1 -> Sum2/2
  Demux/1 -> Sum/1  "e_a"
  Demux/2 -> Sum1/1  "e_b"
  Demux/3 -> Sum2/1  "e_c"
  Subsystem/2(e) -> Demux/1  "e_abc"
  Sum/1 -> Transfer Fcn/1
  Sum1/1 -> Transfer Fcn1/1
  Sum2/1 -> Transfer Fcn2/1
  Transfer Fcn2/1 -> Mux/3  "i_c"
  Transfer Fcn1/1 -> Mux/2  "i_b"
  Transfer Fcn/1 -> Mux/1  "i_a"
  Subsystem/1(e/omega_r) -> f_abc^T*i_abc/1  "f_abc"
  Sum3/1 -> Gain2/1
  f_abc^T*i_abc/1 -> Back-EMF constant/1
  Back-EMF constant/1 -> Pole pairs/1
  t_l/1 -> Sum3/1
  Gain2/1 -> Integrator/1  "alpha_r"
  Integrator/1 -> Subsystem/1(omega_r), omega_r/1, Integrator1/1  "omega_r"
  Integrator1/1 -> Subsystem/2(theta_r), theta_r/1  "theta_r"
  Pole pairs/1 -> t_e/1, Sum3/2  "t_e"
  Mux/1 -> f_abc^T*i_abc/2, i_m/1  "i_abc"

== system CDPR_simulation/Motor 3/FOC BLDC/Direct current controller ==
  error : Inport
  Gain : Gain  Gain=100
  Gain1 : Gain  Gain=70
  Integrator : Integrator
  Sum : Sum  Inputs=++|
  I_d_d : Outport
  wires:
  error/1 -> Gain/1, Integrator/1
  Integrator/1 -> Gain1/1
  Gain1/1 -> Sum/2
  Gain/1 -> Sum/1
  Sum/1 -> I_d_d/1

== system CDPR_simulation/Motor 3/FOC BLDC/Quadrature current controller ==
  error : Inport
  Gain : Gain  Gain=35
  Gain1 : Gain  Gain=50
  Integrator : Integrator
  Sum : Sum  Inputs=++|
  I_q_d : Outport
  wires:
  Sum/1 -> I_q_d/1
  Gain/1 -> Sum/1
  Gain1/1 -> Sum/2
  Integrator/1 -> Gain1/1
  error/1 -> Integrator/1, Gain/1

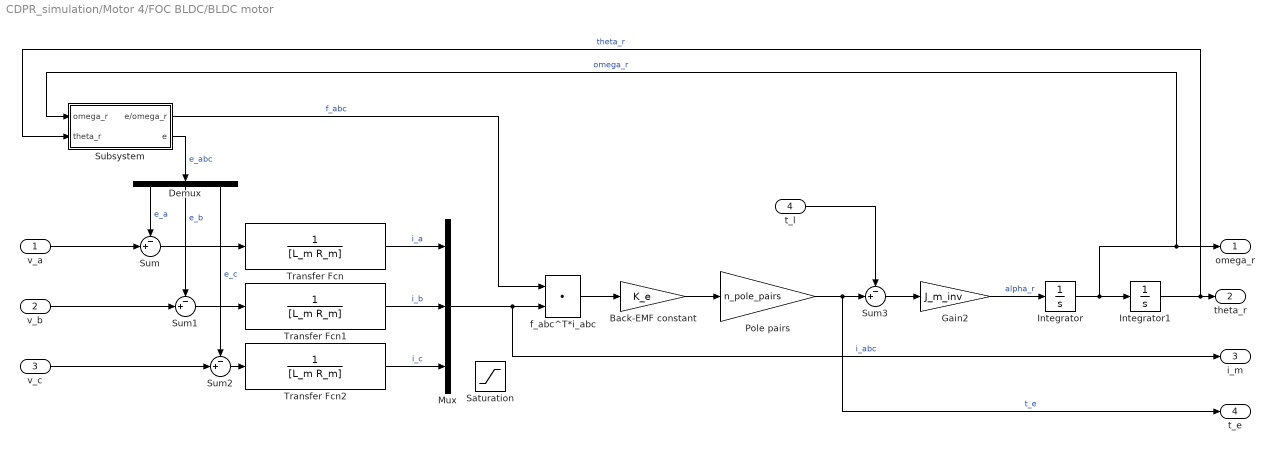
== system CDPR_simulation/Motor 4/FOC BLDC/BLDC motor ==
  v_a : Inport
  v_b : Inport  Port=2
  v_c : Inport  Port=3
  t_l : Inport  Port=4
  Back-EMF constant : Gain  Gain=K_e
  Demux : Demux  Outputs=3
  Gain2 : Gain  Gain=J_m_inv
  Integrator : Integrator  InitialCondition=0.001
  Integrator1 : Integrator  InitialCondition=theta_r_0(4)
  Mux : Mux  Inputs=3
  Pole pairs : Gain  Gain=n_pole_pairs
  Saturation : Saturate  UpperLimit=20  LowerLimit=20
  Subsystem : Subsystem
  Sum{,1..3} (4 alike) : Sum  Inputs=-+|
  Transfer Fcn : TransferFcn  Denominator=[L_m R_m]
  Transfer Fcn1 : TransferFcn  Denominator=[L_m R_m]
  Transfer Fcn2 : TransferFcn  Denominator=[L_m R_m]
  f_abc^T*i_abc : DotProduct  InputSameDT=on  OutDataTypeStr=Inherit: Inherit via internal rule
  omega_r : Outport
  theta_r : Outport  Port=2
  i_m : Outport  Port=3
  t_e : Outport  Port=4
  wires:
  Mux/1 -> i_m/1, f_abc^T*i_abc/2  "i_abc"
  Pole pairs/1 -> Sum3/2, t_e/1  "t_e"
  Integrator1/1 -> theta_r/1, Subsystem/2(theta_r)  "theta_r"
  Integrator/1 -> Integrator1/1, omega_r/1, Subsystem/1(omega_r)  "omega_r"
  Gain2/1 -> Integrator/1  "alpha_r"
  t_l/1 -> Sum3/1
  Back-EMF constant/1 -> Pole pairs/1
  f_abc^T*i_abc/1 -> Back-EMF constant/1
  Sum3/1 -> Gain2/1
  Subsystem/1(e/omega_r) -> f_abc^T*i_abc/1  "f_abc"
  Transfer Fcn/1 -> Mux/1  "i_a"
  Transfer Fcn1/1 -> Mux/2  "i_b"
  Transfer Fcn2/1 -> Mux/3  "i_c"
  Sum2/1 -> Transfer Fcn2/1
  Sum1/1 -> Transfer Fcn1/1
  Sum/1 -> Transfer Fcn/1
  Subsystem/2(e) -> Demux/1  "e_abc"
  Demux/3 -> Sum2/1  "e_c"
  Demux/2 -> Sum1/1  "e_b"
  Demux/1 -> Sum/1  "e_a"
  v_c/1 -> Sum2/2
  v_b/1 -> Sum1/2
  v_a/1 -> Sum/2

== system CDPR_simulation/Motor 4/FOC BLDC/Direct current controller ==
  error : Inport
  Gain : Gain  Gain=100
  Gain1 : Gain  Gain=70
  Integrator : Integrator
  Sum : Sum  Inputs=++|
  I_d_d : Outport
  wires:
  Sum/1 -> I_d_d/1
  Gain/1 -> Sum/1
  Gain1/1 -> Sum/2
  Integrator/1 -> Gain1/1
  error/1 -> Integrator/1, Gain/1

== system CDPR_simulation/Motor 4/FOC BLDC/Quadrature current controller ==
  error : Inport
  Gain : Gain  Gain=35
  Gain1 : Gain  Gain=50
  Integrator : Integrator
  Sum : Sum  Inputs=++|
  I_q_d : Outport
  wires:
  error/1 -> Gain/1, Integrator/1
  Integrator/1 -> Gain1/1
  Gain1/1 -> Sum/2
  Gain/1 -> Sum/1
  Sum/1 -> I_q_d/1

== system CDPR_simulation/Motor 1/FOC BLDC/BLDC motor/Subsystem ==
  omega_r : Inport
  theta_r : Inport  Port=2
  Constant : Constant  Value=fourier_coeff_a
  Constant1 : Constant  Value=fourier_coeff_b
  Gain : Gain  Gain=K_e
  MATLAB Function : MATLAB Function  TreatAsAtomicUnit=on
  Matrix Multiply : Product  Multiplication=Matrix(*)
  e/omega_r : Outport
  e : Outport  Port=2
  wires:
  theta_r/1 -> MATLAB Function/3(theta_r)
  Constant/1 -> MATLAB Function/1(a_f)
  Constant1/1 -> MATLAB Function/2(b_f)
  MATLAB Function/1(f_abc) -> Gain/1
  Gain/1 -> e/omega_r/1, Matrix Multiply/1
  omega_r/1 -> Matrix Multiply/2
  Matrix Multiply/1 -> e/1

== system CDPR_simulation/Motor 2/FOC BLDC/BLDC motor/Subsystem ==
  omega_r : Inport
  theta_r : Inport  Port=2
  Constant : Constant  Value=fourier_coeff_a
  Constant1 : Constant  Value=fourier_coeff_b
  Gain : Gain  Gain=K_e
  MATLAB Function : MATLAB Function  TreatAsAtomicUnit=on
  Matrix Multiply : Product  Multiplication=Matrix(*)
  e/omega_r : Outport
  e : Outport  Port=2
  wires:
  Matrix Multiply/1 -> e/1
  omega_r/1 -> Matrix Multiply/2
  Gain/1 -> Matrix Multiply/1, e/omega_r/1
  MATLAB Function/1(f_abc) -> Gain/1
  Constant1/1 -> MATLAB Function/2(b_f)
  Constant/1 -> MATLAB Function/1(a_f)
  theta_r/1 -> MATLAB Function/3(theta_r)

== system CDPR_simulation/Motor 3/FOC BLDC/BLDC motor/Subsystem ==
  omega_r : Inport
  theta_r : Inport  Port=2
  Constant : Constant  Value=fourier_coeff_a
  Constant1 : Constant  Value=fourier_coeff_b
  Gain : Gain  Gain=K_e
  MATLAB Function : MATLAB Function  TreatAsAtomicUnit=on
  Matrix Multiply : Product  Multiplication=Matrix(*)
  e/omega_r : Outport
  e : Outport  Port=2
  wires:
  theta_r/1 -> MATLAB Function/3(theta_r)
  Constant/1 -> MATLAB Function/1(a_f)
  Constant1/1 -> MATLAB Function/2(b_f)
  MATLAB Function/1(f_abc) -> Gain/1
  Gain/1 -> e/omega_r/1, Matrix Multiply/1
  omega_r/1 -> Matrix Multiply/2
  Matrix Multiply/1 -> e/1

== system CDPR_simulation/Motor 4/FOC BLDC/BLDC motor/Subsystem ==
  omega_r : Inport
  theta_r : Inport  Port=2
  Constant : Constant  Value=fourier_coeff_a
  Constant1 : Constant  Value=fourier_coeff_b
  Gain : Gain  Gain=K_e
  MATLAB Function : MATLAB Function  TreatAsAtomicUnit=on
  Matrix Multiply : Product  Multiplication=Matrix(*)
  e/omega_r : Outport
  e : Outport  Port=2
  wires:
  Matrix Multiply/1 -> e/1
  omega_r/1 -> Matrix Multiply/2
  Gain/1 -> Matrix Multiply/1, e/omega_r/1
  MATLAB Function/1(f_abc) -> Gain/1
  Constant1/1 -> MATLAB Function/2(b_f)
  Constant/1 -> MATLAB Function/1(a_f)
  theta_r/1 -> MATLAB Function/3(theta_r)

== matlab function CDPR_simulation/Motor 2/FOC BLDC/Inverse Park transformation ==
  data: v_q input; v_d input; v_a output; theta_r input; v_b output; v_c output
function [v_a, v_b, v_c] = inverse_park(v_q, v_d, theta_r)
Park_inv = [cos(theta_r)          -sin(theta_r);
            cos(theta_r - 2*pi/3) -sin(theta_r - 2*pi/3);
            cos(theta_r + 2*pi/3) -sin(theta_r + 2*pi/3)];

v_abc = Park_inv*[v_d;v_q];

v_a = v_abc(1);
v_b = v_abc(2);
v_c = v_abc(3);

== matlab function CDPR_simulation/Motor 2/FOC BLDC/Park transformation ==
  data: i_alphabeta input; i_qd output; theta_r input
function i_qd = park(i_alphabeta, theta_r)
Park = [-sin(theta_r) cos(theta_r);
         cos(theta_r) sin(theta_r)];
i_qd = Park*i_alphabeta;

== matlab function CDPR_simulation/Motor 3/FOC BLDC/BLDC motor/Subsystem/MATLAB Function ==
  data: a_f input; f_abc output; b_f input; theta_r input
function f_abc  = normalized_back_EMF(a_f,b_f,theta_r)
sa = 0;
sb = 0;
sc = 0;
ca = 0;
cb = 0;
cc = 0;
n = size(a_f,1);

for i = 1:n
%     ca = ca + a(i,1)*cos((i-1)*theta_r);
    cb = cb + a_f(i,2)*cos((i-1)*theta_r);
    cc = cc + a_f(i,3)*cos((i-1)*theta_r); 
end
for i = 1:2:n
    sa = sa + b_f(i,1)*sin(i*theta_r);
    sb = sb + b_f(i,2)*sin(i*theta_r);
    sc = sc + b_f(i,3)*sin(i*theta_r);
end
f_a = ca+sa;
f_b = cb+sb;
f_c = cc+sc;

f_abc = [f_a;f_b;f_c];

== matlab function CDPR_simulation/Motor 3/FOC BLDC/Inverse Park transformation ==
  data: v_q input; v_d input; v_a output; theta_r input; v_b output; v_c output
function [v_a, v_b, v_c] = inverse_park(v_q, v_d, theta_r)
Park_inv = [cos(theta_r)          -sin(theta_r);
            cos(theta_r - 2*pi/3) -sin(theta_r - 2*pi/3);
            cos(theta_r + 2*pi/3) -sin(theta_r + 2*pi/3)];

v_abc = Park_inv*[v_d;v_q];

v_a = v_abc(1);
v_b = v_abc(2);
v_c = v_abc(3);

== matlab function CDPR_simulation/Motor 3/FOC BLDC/Park transformation ==
  data: i_alphabeta input; i_qd output; theta_r input
function i_qd = park(i_alphabeta, theta_r)
Park = [-sin(theta_r) cos(theta_r);
         cos(theta_r) sin(theta_r)];
i_qd = Park*i_alphabeta;

== matlab function CDPR_simulation/Structure matrix/MATLAB Function ==
  data: a input; u output; b input; pose input; l_ik input; m input
function u = calculateCableUnitVectors(a, b, pose, l_ik, m)
    r = pose(1:2);
    theta = pose(3);
    l = a - r - R_z(theta)*b;
    u = zeros(2,4);
    for i=1:m
        u(:,i) = l(:,i)/l_ik(i);
    end
end

function R = R_z(theta)
    R = [cos(theta) -sin(theta);
         sin(theta)  cos(theta)];
end

== matlab function CDPR_simulation/Motor 4/FOC BLDC/BLDC motor/Subsystem/MATLAB Function ==
  data: a_f input; f_abc output; b_f input; theta_r input
function f_abc  = normalized_back_EMF(a_f,b_f,theta_r)
sa = 0;
sb = 0;
sc = 0;
ca = 0;
cb = 0;
cc = 0;
n = size(a_f,1);

for i = 1:n
%     ca = ca + a(i,1)*cos((i-1)*theta_r);
    cb = cb + a_f(i,2)*cos((i-1)*theta_r);
    cc = cc + a_f(i,3)*cos((i-1)*theta_r); 
end
for i = 1:2:n
    sa = sa + b_f(i,1)*sin(i*theta_r);
    sb = sb + b_f(i,2)*sin(i*theta_r);
    sc = sc + b_f(i,3)*sin(i*theta_r);
end
f_a = ca+sa;
f_b = cb+sb;
f_c = cc+sc;

f_abc = [f_a;f_b;f_c];

== matlab function CDPR_simulation/Motor 4/FOC BLDC/Inverse Park transformation ==
  data: v_q input; v_d input; v_a output; theta_r input; v_b output; v_c output
function [v_a, v_b, v_c] = inverse_park(v_q, v_d, theta_r)
Park_inv = [cos(theta_r)          -sin(theta_r);
            cos(theta_r - 2*pi/3) -sin(theta_r - 2*pi/3);
            cos(theta_r + 2*pi/3) -sin(theta_r + 2*pi/3)];

v_abc = Park_inv*[v_d;v_q];

v_a = v_abc(1);
v_b = v_abc(2);
v_c = v_abc(3);

== matlab function CDPR_simulation/Motor 4/FOC BLDC/Park transformation ==
  data: i_alphabeta input; i_qd output; theta_r input
function i_qd = park(i_alphabeta, theta_r)
Park = [-sin(theta_r) cos(theta_r);
         cos(theta_r) sin(theta_r)];
i_qd = Park*i_alphabeta;

== matlab function CDPR_simulation/Forward kinematics/MATLAB Function ==
  data: a input; y_i output; b input; y_0 input; l input; tau input; epsilon_1 input; epsilon_2 input; xi input; m input
function y_i = MarLevPoseEstimation(a, b, y_0, l, ...
                                    tau, epsilon_1, epsilon_2, xi, ...
                                    m)
    y_i = y_0;
    
    m = size(a, 2);
    
    J = Jacobian(a, b, y_i, l, 1);
    A = J.'*J;
    phi = getPhi(a, b, y_i, l, m);
    g = J.'*phi;
    
    
%     tau       = 1e-6;
    mu        = tau*max(diag(A));
%     epsilon_1 = 1e-17;
%     epsilon_2 = 1e-17;
%     xi        = 2;
    
    iter = 0;
    max_iter = 100;
    
    stop = false;
    while ~stop && iter < max_iter
        iter = iter+1;
    
        h = (A + mu*eye(3))\(-g);
        
        if norm(h,2) <= epsilon_2*(norm(y_i,2)+epsilon_2)
            stop = true;
%             disp(epsilon_2*(norm(y_i,2)+epsilon_2));
%             disp('Stopping algorithm')
        else
            y_new = y_i + h;
    
            % Gain ratio
            Phi = 0.5*(phi.')*phi;
            phi_x_plus_h = getPhi(a, b, y_new, l, m);
            
            Phi_x_plus_h = 0.5*(phi_x_plus_h.')*phi_x_plus_h;
            rho = (Phi - Phi_x_plus_h)/(0.5*(h.')*(mu*h - g));
    
            if rho > 0
                y_i = y_new;
                J = Jacobian(a, b, y_i, l, 1);
                A = J.'*J;
                phi = getPhi(a, b, y_i, l, m);
                g = J.'*phi;
                cond = norm(g,2) < epsilon_1;
                if cond
%                     disp('Stopping algorithm 2')
                    stop = cond;
                end
                mu = mu*max([1/3, 1-(2*rho-1)^3]);
                xi = 2;
            else
                mu = mu*xi;
                xi = 2*xi;
            end
        end
    end
end

function phi = getPhi(a, b, y, l, k_spring, m)
    phi = zeros(4,1);
    for i = 1:size(phi,1)
        phi(i) = nuSquared(a(:,i), b(:,i), y(:), l(i), k_spring);
    end
end

function nuSquared = nuSquared(a, b, y, l, k_spring)
    nuSquared = ...
        k_spring*( ...
              (a(1) - y(1) - b(1)*cos(y(3)) + b(2)*sin(y(3)))^2 ...
            + (y(2) - a(2) + b(2)*cos(y(3)) + b(1)*sin(y(3)))^2 ...
            - l^2 ...
        )^2;
end


function J = Jacobian(a, b, yvec, lvec, k_spring)
    n = size(yvec,1);
    m = size(a,2);

    J = zeros(m,n);
    for i=1:m

        ax = a(1,i);
        ay = a(2,i);
        bx = b(1,i);
        by = b(2,i);
        x     = yvec(1);
        y     = yvec(2);
        theta = yvec(3);
        l = lvec(i);

        k_spring = 1;
        J_x = ...
        -2*k_spring*(    (ax - x - bx*cos(theta) + by*sin(theta))^2        ...
                     +   (y - ay + by*cos(theta) + bx*sin(theta))^2 - l^2) ...
                     * 2*(ax - x - bx*cos(theta) + by*sin(theta));
     
        J_y = ...
         2*k_spring*(   (ax - x - bx*cos(theta) + by*sin(theta))^2         ...
                     +  (y - ay + by*cos(theta) + bx*sin(theta))^2 - l^2)  ...
                     *2*(y - ay + by*cos(theta) + bx*sin(theta));
     
        J_theta = ...
         2*k_spring*(  2*(by*cos(theta) + bx*sin(theta))                   ...
                        *(ax - x - bx*cos(theta) + by*sin(theta))          ...
                     + 2*(bx*cos(theta) - by*sin(theta))                   ...
                        *(y - ay + by*cos(theta) + bx*sin(theta)))         ...
                       *((ax - x - bx*cos(theta) + by*sin(theta))^2        ...
                       + (y - ay + by*cos(theta) + bx*sin(theta))^2 - l^2);
        J(i,:) = [J_x J_y J_theta];
    end
end

== matlab function CDPR_simulation/Forward kinematics/MATLAB Function1 ==
  data: a input; y_0 output; b input; l input
function y_0 = initialPoseEstimate(a, b, l)
    m = size(a,2);
    r_low_i  = zeros(2, m);
    r_high_i = zeros(2, m);
    
    for i=1:m
        r_low_i(:, i)  = ...
            a(:,i) - (l(i) + norm(b(:,i), 2))*[1;1];
        r_high_i(:, i) = ...
            a(:,i) + (l(i) + norm(b(:,i), 2))*[1;1];
    end
    
    r_low = [max(r_low_i(1,:)); 
             max(r_low_i(2,:))];
    
    r_high = [min(r_high_i(1,:));
              min(r_high_i(2,:));];
    
    r_0 = [0.5*(r_low(1) + r_high(1)); 
           0.5*(r_low(2) + r_high(2))];
    y_0 = [r_0; 0.0];
end

== matlab function CDPR_simulation/Inverse kinematics1/Inverse kinematics ==
  data: a input; l output; b input; pose input; m input
function l = inverseKinematics(a, b, pose, m)
    x     = pose(1);
    y     = pose(2);
    theta = pose(3);

    l = zeros(4,1);
    for i=1:m
        l(i) = norm(a(:,i)-[x;y]-R_z(theta)*b(:,i),2);
    end
end


function R = R_z(theta)
    R = [cos(theta) -sin(theta);
         sin(theta)  cos(theta)];
end
